simulink model "problem1_model"  (R2023b)
settings: Solver=FixedStepDiscrete  StartTime=0.0  StopTime=20  FixedStep=0.1  RelTol=1e-3
settings Model: Creator=mluser
settings ModelReferenceCC: EnableRefExpFcnMdlSchedulingChecks=on

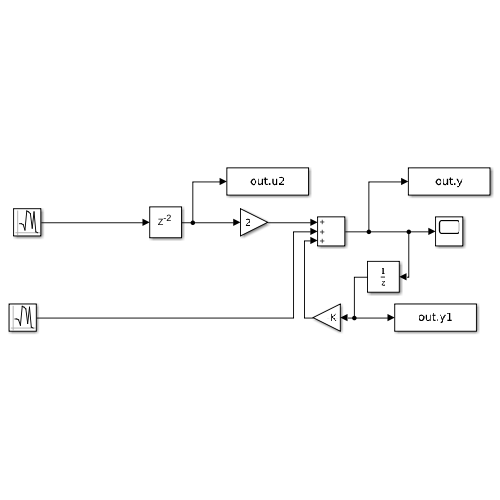
[thumbnail: Simulink's stored preview of the top-level diagram]
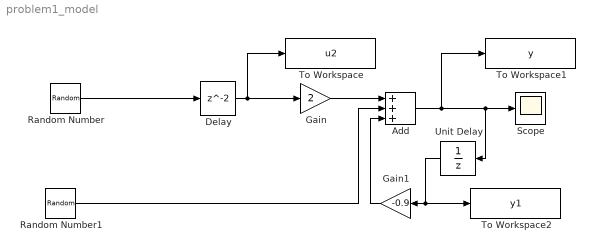
== system problem1_model ==
  Add : Sum  Inputs=+++
  Delay : Delay
  Gain : Gain  Gain=2
  Gain1 : Gain  Gain=-0.9
  Random Number : RandomNumber  SampleTime=0.1
  Random Number1 : RandomNumber  Variance=0.1  SampleTime=0.1
  Scope : Scope
  To Workspace : ToWorkspace  VariableName=u2  SampleTime=-1
  To Workspace1 : ToWorkspace  VariableName=y  SampleTime=-1
  To Workspace2 : ToWorkspace  VariableName=y1  SampleTime=-1
  Unit Delay : UnitDelay  SampleTime=-1  HasFrameUpgradeWarning=on
  wires:
  Random Number/1 -> Delay/1
  Delay/1 -> To Workspace/1, Gain/1
  Gain/1 -> Add/1
  Random Number1/1 -> Add/2
  Add/1 -> To Workspace1/1, Unit Delay/1, Scope/1
  Unit Delay/1 -> To Workspace2/1, Gain1/1
  Gain1/1 -> Add/3
